simulink model "fuzzy2X2MPPT"  (R2023b)
settings: Solver=VariableStepAuto  StartTime=0.0  StopTime=10.0  RelTol=1e-3
libraries: spsDiodeLib x4, spsPVArrayLib x4, spsSeriesRLCBranchLib x4, spsCurrentMeasurementLib x1, fuzblock x1, spsMosfetLib x1, spsPWMGeneratorDCDCLib x1, spsVoltageMeasurementLib x1, spspowerguiLib x1
settings Model: Creator=ASUS  LastModifiedBy=ASUS

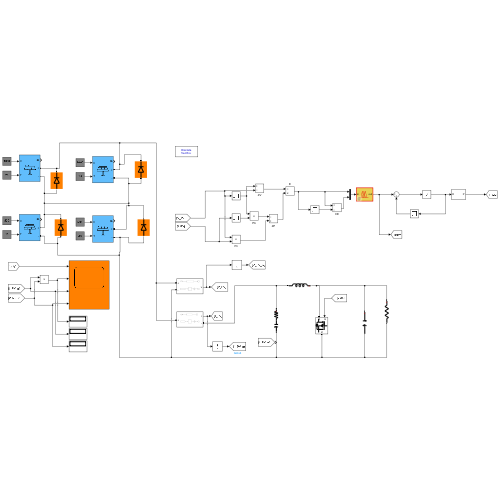
[thumbnail: Simulink's stored preview of the top-level diagram]
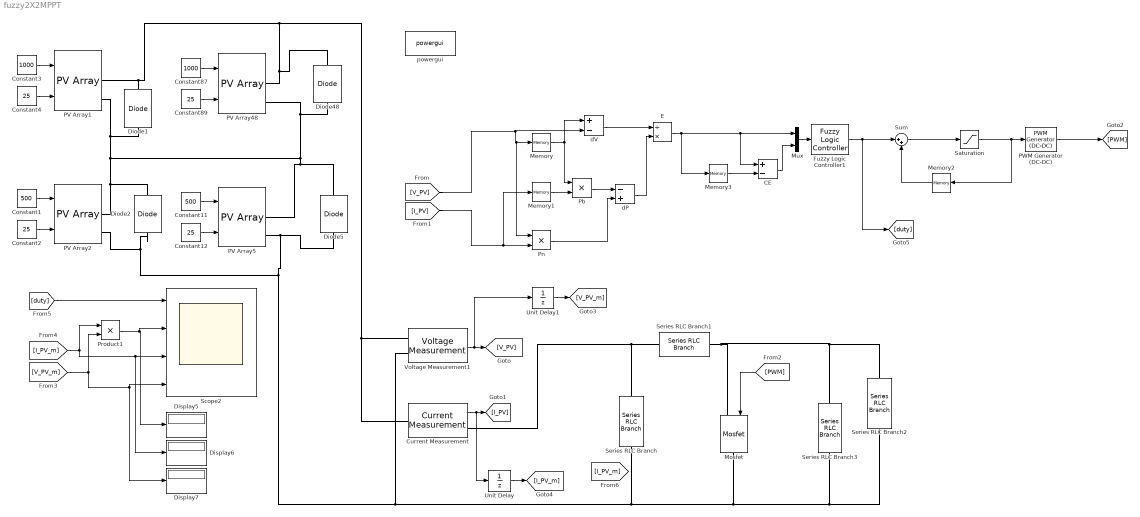
== system fuzzy2X2MPPT ==
  CE : Sum  Inputs=+-
  Constant1 : Constant  Value=500
  Constant11 : Constant  Value=500
  Constant{2,4,12,89} (4 alike) : Constant  Value=25
  Constant3 : Constant  Value=1000
  Constant87 : Constant  Value=1000
  Current Measurement : spsCurrentMeasurementLib/Current Measurement  PhasorSimulation=off  OutputType=Complex  PSBequivalent=0
  Diode{1..2,5,48} (4 alike) : spsDiodeLib/Diode  Ron=0.001  Lon=0  Vf=0.8  IC=0  UseSnubber=0  Rs=inf  Cs=0  Measurements=off
  Display5 : Display
  Display6 : Display
  Display7 : Display
  E : Product  Inputs=/*
  Fuzzy Logic Controller1 : fuzblock/Fuzzy Logic  Controller  FIS='mppt.fis'  OutputSampleNumber=101  DataType=double  FuzzifiedInputs=off  RuleFiringStrengths=off  RuleOutputs=off  AggregatedOutputs=off  SimulateUsing=Interpreted execution  OutOfRangeInputValueMessage=warning  NoRuleFiredMessage=warning  EmptyOutputFuzzySetMessage=warning
  Memory{,1..3} (4 alike) : Memory  InheritSampleTime=on
  Mosfet : spsMosfetLib/Mosfet  Ron=0.1  Lon=0  Rd=0.01  Vfd=0  IC=0  Rs=1e5  Cs=inf  Measurements=off
  Mux : Mux  Inputs=2
  PV Array{1..2,5,48} (4 alike) : spsPVArrayLib/PV Array  Npar=1  Nser=1  PlotType=one module @ 25 deg.C & specified irradiances  S_vec="[ 1000  500  100 ]"  Temp_C_vec="[ 45 25  ]"  ModuleName=BIPV BIPV054-S86  PlotWhenSelected=off  Pm=53.976  Ncell=14  Voc=8.87  Isc=8.22  Vm=6.92  Im=7.8  beta_Voc_pc=-0.36  alpha_Isc_pc=0.06  beta_Voc=-0.031932  alpha_Isc=0.004932  IL=8.263  I0=2.8018e-10  nI=1.0231  Rsh=333.8433  Rs=0.11548  RobustModel=off  RobustCellTemperature=313.3991  BAL=off  Tc=1e-6  Tfilter=5e-5
  PWM Generator (DC-DC) : spsPWMGeneratorDCDCLib/PWM Generator (DC-DC)  Fsw=10000  Ts=0
  Pb : Product
  Pn : Product
  Product1 : Product
  Saturation : Saturate  UpperLimit=0.9  LowerLimit=0.1
  Scope2 : Scope  NumInputPorts=4
  Series RLC Branch : spsSeriesRLCBranchLib/Series RLC Branch  LConnTagsString=__new0  RConnTagsString=__new0  BranchType=RC  Resistance=0.0001  Inductance=1e-3  SetiL0=off  InitialCurrent=0  Capacitance=968e-6  Setx0=off  InitialVoltage=0  Measurements=None
  Series RLC Branch1 : spsSeriesRLCBranchLib/Series RLC Branch  LConnTagsString=__new0  RConnTagsString=__new0  BranchType=L  Resistance=0.0001  Inductance=1.6e-3  SetiL0=off  InitialCurrent=0  Capacitance=968e-6  Setx0=off  InitialVoltage=0  Measurements=None
  Series RLC Branch2 : spsSeriesRLCBranchLib/Series RLC Branch  LConnTagsString=__new0  RConnTagsString=__new0  BranchType=R  Resistance=4  Inductance=1e-3  SetiL0=off  InitialCurrent=0  Capacitance=968e-6  Setx0=off  InitialVoltage=0  Measurements=None
  Series RLC Branch3 : spsSeriesRLCBranchLib/Series RLC Branch  LConnTagsString=__new0  RConnTagsString=__new0  BranchType=C  Resistance=0.0001  Inductance=1e-3  SetiL0=off  InitialCurrent=0  Capacitance=3300e-6  Setx0=off  InitialVoltage=0  Measurements=None
  Sum : Sum  Inputs=|++
  Unit Delay : UnitDelay  SampleTime=-1  HasFrameUpgradeWarning=on
  Unit Delay1 : UnitDelay  SampleTime=-1  HasFrameUpgradeWarning=on
  Voltage Measurement1 : spsVoltageMeasurementLib/Voltage Measurement  PhasorSimulation=off  OutputType=Complex  PSBequivalent=0
  dP : Sum  Inputs=-+
  dV : Sum  Inputs=+-
  powergui : spspowerguiLib/powergui  Priority=1  SimulationMode=Discrete  SampleTime=5e-6  frequency=60  Iterations=50  frequencyindice=0  Pbase=100e6  ErrMax=1e-4  UnitsV=kV  UnitsW=MW  buscounter=0  FunctionMessages=off  echomessages=off  EnableUseOfTLC=off  CurrentSourceSwitches=off  DisableSnubberDevices=off  DisableRonSwitches=off  DisableVfSwitches=off  DisplayEquations=off  AutomaticDiscreteSolvers=off  SolverType=Tustin/Backward Euler (TBE)  Interpol=off  ExternalGateDelay=off  methode=off  Ts=100  x0status=blocks  SPID=on  SwTol=0  HookPort=off  NonlinearTolerance=1e-4  nMaxIteration=100  ContinueOnMaxIteration=off  RestoreLinks=warning  ResistiveCurrentMeasurement=off  Frange=[0:2:500]  Ylog=off  Xlog=on  ShowGrid=off  save=off  variable=ZData  structure=0  ZoomFFT=off  StartTime=0.0  cycles=1  DisplayStyle=1  fundamental=60  FreqAxis=off  MaxFrequency=1000  frequencyindicesteady=1  RmsSteady=1  display=off
  wires:
  Constant3/1 -> PV Array1/1
  Constant4/1 -> PV Array1/2
  Constant1/1 -> PV Array2/1
  Constant2/1 -> PV Array2/2
  Constant87/1 -> PV Array48/1
  Constant11/1 -> PV Array5/1
  Constant89/1 -> PV Array48/2
  [PWM] -> Mosfet/1
  Constant12/1 -> PV Array5/2
  Fuzzy Logic Controller1/1 -> [duty], Sum/1
  PWM Generator (DC-DC)/1 -> [PWM]
  [I_PV] -> Memory1/1, Pn/2
  E/1 -> Mux/1, CE/1, Memory3/1
  Saturation/1 -> Memory2/1, PWM Generator (DC-DC)/1
  dV/1 -> E/1
  dP/1 -> E/2
  Memory1/1 -> Pb/2
  Sum/1 -> Saturation/1
  CE/1 -> Mux/2
  [V_PV] -> Pn/1, Memory/1, dV/2
  Memory/1 -> dV/1, Pb/1
  Memory2/1 -> Sum/2
  Pb/1 -> dP/1
  Mux/1 -> Fuzzy Logic Controller1/1
  Memory3/1 -> CE/2
  Pn/1 -> dP/2
  [duty] -> Scope2/1
  [V_PV_m] -> Product1/2, Display7/1, Scope2/4
  Product1/1 -> Scope2/2, Display5/1
  [I_PV_m] -> Product1/1, Display6/1, Scope2/3
  Unit Delay1/1 -> [V_PV_m]
  Voltage Measurement1/1 -> Unit Delay1/1, [V_PV]
  Unit Delay/1 -> [I_PV_m]
  Current Measurement/1 -> Unit Delay/1, [I_PV]
  connections:
  PV Array2/RConn1 -- Diode2/RConn1 -- Diode1/LConn1 -- PV Array1/RConn2 -- PV Array48/RConn2 -- Diode48/LConn1 -- PV Array5/RConn1 -- Diode5/RConn1
  PV Array48/RConn1 -- Diode48/RConn1 -- Diode1/RConn1 -- PV Array1/RConn1 -- Voltage Measurement1/LConn1 -- Current Measurement/LConn1
  PV Array5/RConn2 -- Diode5/LConn1 -- Series RLC Branch/RConn1 -- Mosfet/RConn1 -- Series RLC Branch2/RConn1 -- Series RLC Branch3/RConn1 -- Voltage Measurement1/LConn2 -- Diode2/LConn1 -- PV Array2/RConn2
  Series RLC Branch3/LConn1 -- Series RLC Branch2/LConn1 -- Series RLC Branch1/LConn1 -- Mosfet/LConn1
  Series RLC Branch1/RConn1 -- Series RLC Branch/LConn1 -- Current Measurement/RConn1
